simulink model "levitron_sim"  (Simulink 7.1)
settings: Solver=ode4  SolverMode=SingleTasking  StartTime=0.0  StopTime=200  FixedStep=0.01  MaxStep=.01  RelTol=1e-3  AbsTol=1e-6
undefined symbols (not defined in the file): Levitron, levitron_lib
libraries: simulink x2
Description:
  | Bouncing Ball Model: Use of Zero Crossing Detection
  | 
  | A rubber ball is thrown into the air with a velocity of 15
  | meters per second from a height of 10 m.  The position
  | of the ball is shown in the lower plot of the scope, and
  | the velocity of the ball is shown in the upper plot.
  | 
  | This system uses a reset integrator to change the
  | direction of the ball as it comes into contact with
  | the ground, the zero crossing detection prevents the
  | ball from going below the ground.
settings Model: Creator=The MathWorks Inc.  LastModifiedBy=volgy  CovMetricSettings=d  ExtModeTrigMode=oneshot  ExtModeArmWhenConnect=off  ExtModeAutoUpdateStatusClock=off
settings DataIOCC: ExternalInput=[]  InitialState=[]  LimitDataPoints=off  SaveOutput=off  SaveTime=off
settings OptimizationCC: BooleanDataType=off  InlineInvariantSignals=on  BufferReusableBoundary=off
settings DebuggingCC: SaveWithParameterizedLinksMsg=none  SignalResolutionControl=TryResolveAllWithWarning  SolverPrmCheckMsg=none  MultiTaskDSMMsg=warning  MultiTaskCondExecSysMsg=none  SigSpecEnsureSampleTimeMsg=none  BusObjectLabelMismatch=none  StrictBusMsg=None
settings HardwareCC: TargetUnknown=on
settings RTWCC: IncludeERTFirstTime=on
settings CodeAppCC: CustomSymbolStrFcn=$F$N$M
settings GRTTargetCC: TargetFcnLib=ansi_tfl_tmw.mat

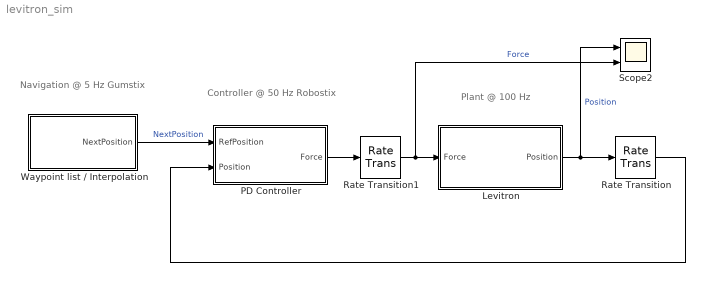
== system levitron_sim ==
  note: Controller @ 50 Hz
      | Robostix
  note: Plant @ 100 Hz
  note: Navigation @ 5 Hz
      | Gumstix
  Levitron : Subsystem  AncestorBlock=levitron_lib/Levitron  mask{mass=1, gravity=-9.81, v0=15, z0=10}
      mask prompts: mass "Mass (g)"; gravity "Gravity (m/s^2)"; v0 "Initial velocity (m/s)"; z0 "Initial position (m)"
  PD Controller : Subsystem  AncestorBlock=levitron_lib/PD Controller
  Rate Transition : RateTransition  OutPortSampleTime=0.02
  Rate Transition1 : RateTransition  OutPortSampleTime=0.01
  Scope2 : Scope  NumInputPorts=2
      settings: YMin=-5~0  YMax=5~50
  Waypoint list / Interpolation : Subsystem  AncestorBlock=levitron_lib/Waypoint list // Interpolation  mask{sample_time=0.2, time_values=[0 20 40 60 80 100], output_values=[10 50 30 20 40 10]}
      mask prompts: sample_time "Sample Time (s)"; time_values "Time Values"; output_values "Output Values"
  wires:
  PD Controller/1(Force) -> Rate Transition1/1
  Rate Transition1/1 -> Levitron/1(Force), Scope2/2  "Force"
  Levitron/1(Position) -> Rate Transition/1, Scope2/1  "Position"
  Waypoint list / Interpolation/1(NextPosition) -> PD Controller/1(RefPosition)  "NextPosition"
  Rate Transition/1 -> PD Controller/2(Position)

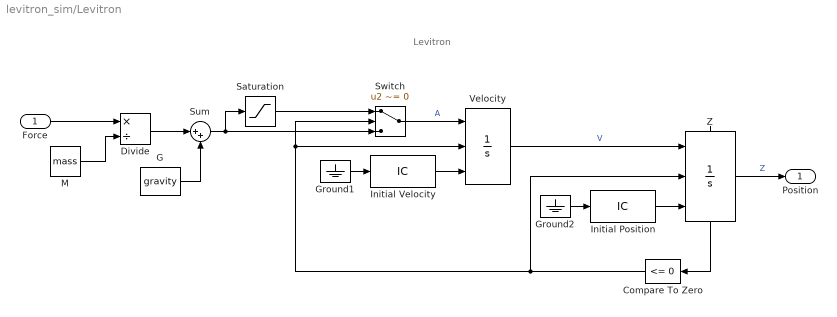
== system levitron_sim/Levitron ==
  note: Levitron
  Force : Inport  OutDataType=sfix(16)  OutScaling=2^0
  Compare To Zero : simulink/Logic and Bit Operations/Compare To Zero  Orientation=left  SystemSampleTime=-1  relop=<=  LogicOutDataTypeMode=boolean
  Divide : Product  Inputs=*/  OutDataType=sfix(16)  OutScaling=2^-10
  G : Constant  Value=gravity  OutDataType=sfix(16)  OutScaling=2^0
  Ground1 : Ground
  Ground2 : Ground
  Initial Position : InitialCondition  Value=z0
  Initial Velocity : InitialCondition  Value=v0
  M : Constant  Value=mass  OutDataType=sfix(16)  OutScaling=2^0
  Saturation : Saturate  UpperLimit=inf  LowerLimit=0.0  OutDataType=sfix(16)  OutScaling=2^0
  Sum : Sum  Inputs=|++  OutDataType=sfix(16)  OutScaling=2^0
  Switch : Switch  Criteria=u2 ~= 0  OutDataType=sfix(16)  OutScaling=2^0
  Velocity : Integrator  ExternalReset=rising  InitialConditionSource=external
  Z : Integrator  ExternalReset=rising  InitialConditionSource=external  InitialCondition=10  LimitOutput=on  LowerSaturationLimit=0  ShowStatePort=on
      settings: AttributesFormatString=Xo = %<InitialCondition>
  Position : Outport  OutDataType=sfix(16)  OutScaling=2^0
  wires:
  Initial Velocity/1 -> Velocity/3
  Velocity/1 -> Z/1  "V"
  Ground2/1 -> Initial Position/1
  Compare To Zero/1 -> Z/2, Switch/2, Velocity/2
  Initial Position/1 -> Z/3
  Z/State -> Compare To Zero/1
  Ground1/1 -> Initial Velocity/1
  Switch/1 -> Velocity/1  "A"
  Saturation/1 -> Switch/1
  Sum/1 -> Switch/3, Saturation/1
  M/1 -> Divide/2
  Divide/1 -> Sum/1
  G/1 -> Sum/2
  Z/1 -> Position/1  "Z"
  Force/1 -> Divide/1

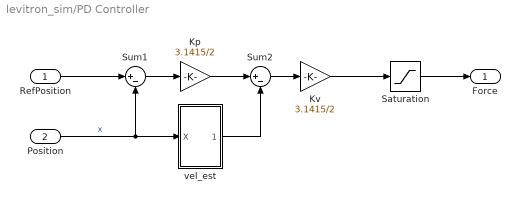
== system levitron_sim/PD Controller ==
  RefPosition : Inport
  Position : Inport  Port=2
  Kp : Gain  Gain=3.1415/2  ParameterDataType=sfix(16)  ParameterScaling=2^0  OutDataType=sfix(16)  OutScaling=2^0
  Kv : Gain  Gain=3.1415/2  ParameterDataType=sfix(16)  ParameterScaling=2^0  OutDataType=sfix(16)  OutScaling=2^0
  Saturation : Saturate  UpperLimit=100  LowerLimit=0  OutDataType=sfix(16)  OutScaling=2^0
  Sum1 : Sum  Inputs=|+-  OutDataType=sfix(16)  OutScaling=2^0
  Sum2 : Sum  Inputs=|+-  OutDataType=sfix(16)  OutScaling=2^0
  vel_est : Subsystem
  Force : Outport
  wires:
  Kv/1 -> Saturation/1
  Sum2/1 -> Kv/1
  vel_est/1(V_est) -> Sum2/2
  Kp/1 -> Sum2/1
  Sum1/1 -> Kp/1
  Saturation/1 -> Force/1
  RefPosition/1 -> Sum1/1
  Position/1 -> Sum1/2, vel_est/1(X)  "x"

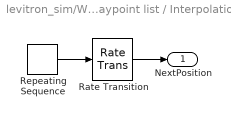
== system levitron_sim/Waypoint list / Interpolation ==
  Rate Transition : RateTransition  OutPortSampleTime=sample_time
  Repeating Sequence : simulink/Sources/Repeating Sequence  SystemSampleTime=-1  rep_seq_t=time_values  rep_seq_y=output_values
  NextPosition : Outport
  wires:
  Rate Transition/1 -> NextPosition/1
  Repeating Sequence/1 -> Rate Transition/1

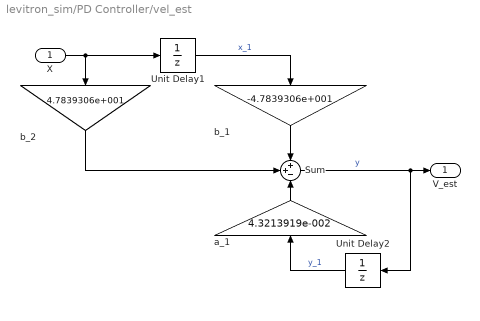
== system levitron_sim/PD Controller/vel_est ==
  X : Inport
  Sum : Sum  Inputs=++-  AccumDataTypeStr=single  OutDataType=sfix(16)  OutScaling=2^0
  Unit Delay1 : UnitDelay  SampleTime=-1
  Unit Delay2 : UnitDelay  Orientation=left  SampleTime=-1
  a_1 : Gain  Orientation=up  Gain=4.3213919e-002  ParameterDataType=sfix(16)  ParameterScaling=2^0  OutDataTypeMode=single  OutDataType=sfix(16)  OutScaling=2^0  OutDataTypeStr=single
  b_1 : Gain  Orientation=down  Gain=-4.7839306e+001  ParameterDataType=sfix(16)  ParameterScaling=2^0  OutDataTypeMode=single  OutDataType=sfix(16)  OutScaling=2^0  OutDataTypeStr=single
  b_2 : Gain  Orientation=down  Gain=4.7839306e+001  ParameterDataType=sfix(16)  ParameterScaling=2^0  OutDataTypeMode=single  OutDataType=sfix(16)  OutScaling=2^0  OutDataTypeStr=single
  V_est : Outport
  wires:
  X/1 -> Unit Delay1/1, b_2/1
  Unit Delay2/1 -> a_1/1  "y_1"
  a_1/1 -> Sum/3
  Sum/1 -> V_est/1, Unit Delay2/1  "y"
  b_2/1 -> Sum/2
  b_1/1 -> Sum/1
  Unit Delay1/1 -> b_1/1  "x_1"
